simulink model "first"  (R2021a)
settings: Solver=FixedStepAuto  StartTime=0.0  StopTime=150  FixedStep=0.1  RelTol=1e-3
(part 1 of 2)
settings Model: Creator=templ  LastModifiedBy=templ
settings DataIOCC: ReturnWorkspaceOutputs=off

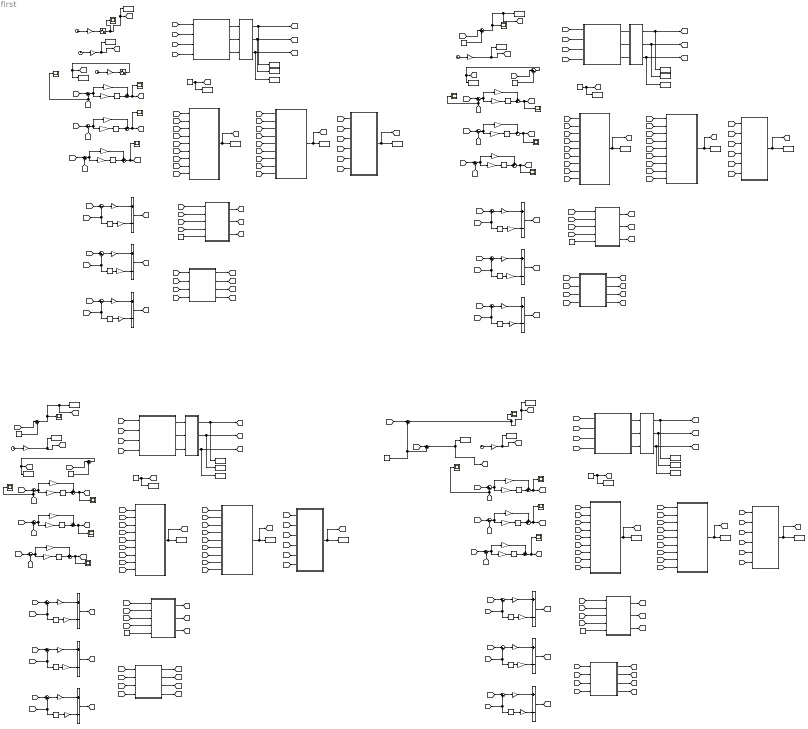
== system first ==
  note: Attitude
  note: Position
  note: Attitude
  note: Position
  note: Attitude
  note: Position
  note: Position
  note: Attitude
  Add{,1..11} (12 alike) : Sum  Inputs=+-
  Attitude Control Module : Subsystem
  Attitude Control Module1 : Subsystem
  Attitude Control Module2 : Subsystem
  Attitude Control Module3 : Subsystem
  Clock{,1..4,7} (6 alike) : Clock
  Constant{,1..4} (5 alike) : Constant  Value=5
  Derivative{,1..23} (24 alike) : Derivative
  Gain{,2,14,20,22,33,41,48} (8 alike) : Gain  Gain=0.03
  Gain{1,3,16,21,23,34,42,49} (8 alike) : Gain  Gain=0.8
  Gain{10,17,30,43} (4 alike) : Gain  Gain=0.25
  Gain{6,8,11,18,26,28,31,37,39,44,52,54} (12 alike) : Gain  Gain=0.5
  Gain{7,9,12..13,27,29,38,40,53,55} (10 alike) : Gain  Gain=0.2
  Gain{15,19,32,47} (4 alike) : Gain  Gain=0.1
  Gain{4,24,35,50} (4 alike) : Gain  Gain=0.05
  Gain{5,25,36,51} (4 alike) : Gain  Gain=0.32
  MATLAB Function : MATLAB Function  TreatAsAtomicUnit=on
  MATLAB Function1 : MATLAB Function  TreatAsAtomicUnit=on
  MATLAB Function2 : MATLAB Function  TreatAsAtomicUnit=on
  MATLAB Function3 : MATLAB Function  TreatAsAtomicUnit=on
  MATLAB Function4 : MATLAB Function  TreatAsAtomicUnit=on
  MATLAB Function5 : MATLAB Function  TreatAsAtomicUnit=on
  MATLAB Function6 : MATLAB Function  TreatAsAtomicUnit=on
  MATLAB Function7 : MATLAB Function  TreatAsAtomicUnit=on
  Position : MATLAB Function  TreatAsAtomicUnit=on
  Position1 : MATLAB Function  TreatAsAtomicUnit=on
  Position2 : MATLAB Function  TreatAsAtomicUnit=on
  Position3 : MATLAB Function  TreatAsAtomicUnit=on
  Scope{,1..19} (20 alike) : Scope
  Sine Wave : Sin  TimeSource=Use external signal  Amplitude=2  SampleTime=0
  Sine Wave Function1 : Sin  TimeSource=Use external signal  Amplitude=2  Phase=pi/2  SampleTime=0
  Subsystem : Subsystem
  Subsystem1 : Subsystem
  Subsystem2 : Subsystem
  Subsystem3 : Subsystem
  Subsystem4 : Subsystem
  Subsystem5 : Subsystem
  Subsystem6 : Subsystem
  Subsystem7 : Subsystem
  Sum{,2,4,6..9,11,13,15..19,21,23,25..27,30..31,33,35,37..39,41} (27 alike) : Sum  Inputs=|+-
  Sum{1,3,5,10,12,14,20,22,24,32,34,36} (12 alike) : Sum  Inputs=++|
  Sum28 : Sum  Inputs=|++
  Sum29 : Sum  Inputs=|++
  Sum40 : Sum  Inputs=|++
  To Workspace : ToWorkspace  VariableName=phi  SampleTime=-1
  To Workspace1 : ToWorkspace  VariableName=theta  SampleTime=-1
  To Workspace10 : ToWorkspace  VariableName=psaid  SampleTime=-1
  To Workspace11 : ToWorkspace  VariableName=theta1  SampleTime=-1
  To Workspace12 : ToWorkspace  VariableName=psaid1  SampleTime=-1
  To Workspace13 : ToWorkspace  VariableName=psai1  SampleTime=-1
  To Workspace14 : ToWorkspace  VariableName=x1  SampleTime=-1
  To Workspace15 : ToWorkspace  VariableName=y1  SampleTime=-1
  To Workspace16 : ToWorkspace  VariableName=z1  SampleTime=-1
  To Workspace17 : ToWorkspace  VariableName=xd1  SampleTime=-1
  To Workspace18 : ToWorkspace  VariableName=yd1  SampleTime=-1
  To Workspace19 : ToWorkspace  VariableName=zd1  SampleTime=-1
  To Workspace2 : ToWorkspace  VariableName=psai  SampleTime=-1
  To Workspace20 : ToWorkspace  VariableName=theta2  SampleTime=-1
  To Workspace21 : ToWorkspace  VariableName=psaid2  SampleTime=-1
  To Workspace22 : ToWorkspace  VariableName=psai2  SampleTime=-1
  To Workspace23 : ToWorkspace  VariableName=x2  SampleTime=-1
  To Workspace24 : ToWorkspace  VariableName=y2  SampleTime=-1
  To Workspace25 : ToWorkspace  VariableName=z2  SampleTime=-1
  To Workspace26 : ToWorkspace  VariableName=xd2  SampleTime=-1
  To Workspace27 : ToWorkspace  VariableName=yd2  SampleTime=-1
  To Workspace28 : ToWorkspace  VariableName=zd2  SampleTime=-1
  To Workspace29 : ToWorkspace  VariableName=phi2  SampleTime=-1
  To Workspace3 : ToWorkspace  VariableName=x  SampleTime=-1
  To Workspace30 : ToWorkspace  VariableName=phi3  SampleTime=-1
  To Workspace31 : ToWorkspace  VariableName=theta3  SampleTime=-1
  To Workspace32 : ToWorkspace  VariableName=psaid3  SampleTime=-1
  To Workspace33 : ToWorkspace  VariableName=psai3  SampleTime=-1
  To Workspace34 : ToWorkspace  VariableName=x3  SampleTime=-1
  To Workspace35 : ToWorkspace  VariableName=y3  SampleTime=-1
  To Workspace36 : ToWorkspace  VariableName=z3  SampleTime=-1
  To Workspace37 : ToWorkspace  VariableName=xd3  SampleTime=-1
  To Workspace38 : ToWorkspace  VariableName=yd3  SampleTime=-1
  To Workspace39 : ToWorkspace  VariableName=zd3  SampleTime=-1
  To Workspace4 : ToWorkspace  VariableName=y  SampleTime=-1
  To Workspace5 : ToWorkspace  VariableName=z  SampleTime=-1
  To Workspace6 : ToWorkspace  VariableName=xd  SampleTime=-1
  To Workspace7 : ToWorkspace  VariableName=yd  SampleTime=-1
  To Workspace8 : ToWorkspace  VariableName=zd  SampleTime=-1
  To Workspace9 : ToWorkspace  VariableName=phi1  SampleTime=-1
  m{,1..3} (4 alike) : Constant  Value=1.5
  psaid{1..4} (4 alike) : Constant  Value=0.2
  x : Subsystem
  x1 : Subsystem
  x2 : Subsystem
  x3 : Subsystem
  wires:
  Gain12/1 -> Sine Wave/1
  Sine Wave/1 -> Scope2/1, To Workspace6/1, [xd]
  Clock/1 -> Gain12/1
  Clock3/1 -> Gain15/1
  Gain15/1 -> [zd], To Workspace8/1
  Gain13/1 -> Sine Wave Function1/1
  Clock1/1 -> Gain13/1
  Sine Wave Function1/1 -> To Workspace7/1, [yd]
  Gain/1 -> Sum1/1
  Gain1/1 -> Derivative/1
  [x] -> Scope8/1, Sum/2
  Sum1/1 -> Scope/1, [Ux]
  Derivative/1 -> Sum1/2
  Sum/1 -> Gain1/1, Gain/1
  [xd] -> Sum/1
  Sum2/1 -> Gain3/1, Gain2/1
  Gain3/1 -> Derivative1/1
  Gain2/1 -> Sum3/1
  [y] -> Sum2/2
  Derivative1/1 -> Sum3/2
  [yd] -> Sum2/1
  [z] -> Sum4/2
  Sum4/1 -> Gain5/1, Gain4/1
  Gain4/1 -> Sum5/1
  [zd] -> Sum4/1
  Derivative2/1 -> Sum5/2
  Gain5/1 -> Derivative2/1
  [w2] -> Attitude Control Module/2(w2)
  [w1] -> Attitude Control Module/4(w1)
  [w3] -> Attitude Control Module/3(w3)
  MATLAB Function1/1(phi) -> To Workspace/1, [phi]
  MATLAB Function1/2(theta) -> To Workspace1/1, [theta]
  MATLAB Function1/3(psai) -> To Workspace2/1, [psai]
  Attitude Control Module/3(psai) -> MATLAB Function1/3(u3)
  Attitude Control Module/2(theta) -> MATLAB Function1/2(u2)
  Attitude Control Module/1(phi) -> MATLAB Function1/1(u1)
  [w4] -> Attitude Control Module/1(w4)
  [w4] -> Subsystem1/3(In3)
  [phi] -> Subsystem1/1(In1)
  [w3] -> Subsystem1/5(In5)
  [psai] -> Subsystem/3(In3)
  [theta] -> Subsystem/2(In2)
  [psai] -> x/3(In3)
  [w2] -> x/7(In7)
  [w4] -> x/6(In6)
  [theta] -> Subsystem1/2(In2)
  [phi] -> x/4(In4)
  [psai] -> x/5(In5)
  [w3] -> x/8(In8)
  [phi] -> Subsystem/4(In4)
  [w1] -> Subsystem1/6(In6)
  [w1] -> x/9(In9)
  [w1] -> Subsystem/9(In9)
  [psai] -> Subsystem/5(In5)
  [theta] -> x/2(In2)
  [w2] -> Subsystem/7(In7)
  [w4] -> Subsystem/6(In6)
  Subsystem1/1(Out1) -> [z], To Workspace5/1
  [w2] -> Subsystem1/4(In4)
  Subsystem/1(Out1) -> [y], To Workspace4/1
  [w3] -> Subsystem/8(In8)
  [phi] -> Subsystem/1(In1)
  x/1(Out1) -> [x], To Workspace3/1
  [phi] -> x/1(In1)
  Position/2(phid) -> [phid]
  Position/1(U1) -> [U1]
  [Uy] -> Position/2(Uy)
  [Ux] -> Position/1(Ux)
  m/1 -> Position/5(m)
  [psaid] -> Position/4(psaid)
  Position/3(thetad) -> [thetad]
  [Uz] -> Position/3(Uz)
  Gain7/1 -> Add/2
  Derivative3/1 -> Gain7/1
  [phid] -> Sum6/1
  [phi] -> Derivative3/1, Sum6/2
  Add/1 -> [U2]
  Gain6/1 -> Add/1
  Sum6/1 -> Gain6/1
  [theta] -> Derivative4/1, Sum7/2
  [thetad] -> Sum7/1
  Gain8/1 -> Add1/1
  Gain9/1 -> Add1/2
  Sum7/1 -> Gain8/1
  Derivative4/1 -> Gain9/1
  Add1/1 -> [U3]
  Derivative5/1 -> Gain11/1
  [psaid] -> Sum8/1
  Sum8/1 -> Gain10/1
  Gain10/1 -> Add2/1
  [psai] -> Derivative5/1, Sum8/2
  Add2/1 -> [U4]
  Gain11/1 -> Add2/2
  MATLAB Function/2(w2) -> [w2]
  MATLAB Function/3(w3) -> [w3]
  MATLAB Function/4(w4) -> [w4]
  MATLAB Function/1(w1) -> [w1]
  [U1] -> MATLAB Function/1(U1)
  [U3] -> MATLAB Function/3(U3)
  [U2] -> MATLAB Function/2(U2)
  [U4] -> MATLAB Function/4(U4)
  psaid1/1 -> To Workspace10/1, [psaid]
  Add4/1 -> [U31]
  Derivative10/1 -> Gain29/1
  Gain29/1 -> Add4/2
  Sum16/1 -> Gain28/1
  [theta1] -> Derivative10/1, Sum16/2
  Gain18/1 -> Add5/2
  Add5/1 -> [U41]
  [psai1] -> Derivative11/1, Sum17/2
  Gain17/1 -> Add5/1
  Sum17/1 -> Gain17/1
  [psaid1] -> Sum17/1
  [w11] -> Subsystem3/6(In6)
  [w21] -> Subsystem3/4(In4)
  Subsystem3/1(Out1) -> [z1], To Workspace16/1
  Derivative11/1 -> Gain18/1
  [w41] -> Subsystem2/6(In6)
  [w21] -> Subsystem2/7(In7)
  [theta1] -> x1/2(In2)
  [psai1] -> Subsystem2/5(In5)
  [w11] -> Subsystem2/9(In9)
  [w11] -> x1/9(In9)
  [phid1] -> Sum15/1
  Derivative9/1 -> Gain27/1
  [phi1] -> Derivative9/1, Sum15/2
  Add3/1 -> [U21]
  [U41] -> MATLAB Function2/4(U4)
  MATLAB Function2/4(w4) -> [w41]
  Gain16/1 -> Derivative6/1
  Gain14/1 -> Sum10/1
  [x1] -> Scope9/1, Sum9/2
  [phi1] -> Subsystem2/4(In4)
  Gain28/1 -> Add4/1
  psaid2/1 -> To Workspace12/1, [psaid1]
  [U21] -> MATLAB Function2/2(U2)
  [U11] -> MATLAB Function2/1(U1)
  [w31] -> x1/8(In8)
  MATLAB Function2/1(w1) -> [w11]
  m1/1 -> Position1/5(m)
  [Uz1] -> Position1/3(Uz)
  Position1/3(thetad) -> [thetad1]
  [psaid1] -> Position1/4(psaid)
  [w41] -> Subsystem3/3(In3)
  [Ux1] -> Position1/1(Ux)
  [xd1] -> Sum9/1
  Sum9/1 -> Gain16/1, Gain14/1
  Derivative6/1 -> Sum10/2
  [w31] -> Attitude Control Module1/3(w3)
  [w11] -> Attitude Control Module1/4(w1)
  MATLAB Function3/3(psai) -> To Workspace13/1, [psai1]
  [w21] -> Attitude Control Module1/2(w2)
  Attitude Control Module1/2(theta) -> MATLAB Function3/2(u2)
  Attitude Control Module1/3(psai) -> MATLAB Function3/3(u3)
  [Uy1] -> Position1/2(Uy)
  Gain27/1 -> Add3/2
  Position1/2(phid) -> [phid1]
  x1/1(Out1) -> [x1], To Workspace14/1
  [phi1] -> Subsystem2/1(In1)
  Gain26/1 -> Add3/1
  [phi1] -> x1/1(In1)
  Derivative8/1 -> Sum14/2
  Subsystem2/1(Out1) -> [y1], To Workspace15/1
  [thetad1] -> Sum16/1
  [zd1] -> Sum13/1
  Gain24/1 -> Sum14/1
  Attitude Control Module1/1(phi) -> MATLAB Function3/1(u1)
  [theta1] -> Subsystem3/2(In2)
  [w41] -> x1/6(In6)
  [U31] -> MATLAB Function2/3(U3)
  [w21] -> x1/7(In7)
  [w41] -> Attitude Control Module1/1(w4)
  MATLAB Function2/3(w3) -> [w31]
  [psai1] -> x1/3(In3)
  [theta1] -> Subsystem2/2(In2)
  [psai1] -> Subsystem2/3(In3)
  [w31] -> Subsystem3/5(In5)
  Sum13/1 -> Gain25/1, Gain24/1
  [psai1] -> x1/5(In5)
  MATLAB Function3/1(phi) -> To Workspace9/1, [phi1]
  [y1] -> Sum11/2
  Gain19/1 -> [zd1], To Workspace19/1
  [phi1] -> Subsystem3/1(In1)
  [w31] -> Subsystem2/8(In8)
  MATLAB Function3/2(theta) -> To Workspace11/1, [theta1]
  [yd1] -> Sum11/1
  Derivative7/1 -> Sum12/2
  Sum11/1 -> Gain23/1, Gain22/1
  [z1] -> Sum13/2
  Gain25/1 -> Derivative8/1
  MATLAB Function2/2(w2) -> [w21]
  [phi1] -> x1/4(In4)
  Gain23/1 -> Derivative7/1
  Position1/1(U1) -> [U11]
  Sum15/1 -> Gain26/1
  Gain22/1 -> Sum12/1
  [xd] -> Sum18/1
  Clock2/1 -> Gain19/1
  Sum3/1 -> Scope3/1, [Uy]
  Sum5/1 -> Scope4/1, [Uz]
  Sum10/1 -> Scope5/1, [Ux1]
  Sum12/1 -> Scope6/1, [Uy1]
  Sum14/1 -> Scope7/1, [Uz1]
  Constant/1 -> Sum18/2
  Sum18/1 -> Scope1/1, [xd1], To Workspace17/1
  Constant1/1 -> Sum19/2
  [yd] -> Sum19/1
  Sum19/1 -> To Workspace18/1, [yd1]
  [yd] -> Sum29/1
  Constant2/1 -> Sum28/2
  Clock4/1 -> Gain32/1
  [xd] -> Sum28/1
  Gain32/1 -> [zd2], To Workspace28/1
  Sum28/1 -> Scope10/1, [xd2], To Workspace26/1
  Sum29/1 -> To Workspace27/1, [yd2]
  [theta2] -> x2/2(In2)
  [w42] -> Subsystem4/6(In6)
  [w22] -> Subsystem5/4(In4)
  Add8/1 -> [U42]
  [psaid2] -> Sum27/1
  Derivative13/1 -> Gain31/1
  [w32] -> x2/8(In8)
  Sum23/1 -> Gain36/1, Gain35/1
  [yd2] -> Sum21/1
  MATLAB Function5/1(phi) -> To Workspace29/1, [phi2]
  [psai2] -> x2/5(In5)
  [phi2] -> x2/1(In1)
  MATLAB Function5/3(psai) -> To Workspace22/1, [psai2]
  [phi2] -> Subsystem5/1(In1)
  [w32] -> Subsystem5/5(In5)
  m2/1 -> Position2/5(m)
  Gain30/1 -> Add8/1
  Add6/1 -> [U22]
  [psai2] -> Subsystem4/3(In3)
  [theta2] -> Derivative12/1, Sum26/2
  [psai2] -> Subsystem4/5(In5)
  [psai2] -> x2/3(In3)
  MATLAB Function4/1(w1) -> [w12]
  [theta2] -> Subsystem4/2(In2)
  Sum24/1 -> Scope13/1, [Uz2]
  [w12] -> Subsystem5/6(In6)
  x2/1(Out1) -> [x2], To Workspace23/1
  [U32] -> MATLAB Function4/3(U3)
  Sum26/1 -> Gain39/1
  Gain38/1 -> Add6/2
  [thetad2] -> Sum26/1
  Sum20/1 -> Scope11/1, [Ux2]
  [psaid2] -> Position2/4(psaid)
  [zd2] -> Sum23/1
  [x2] -> Scope14/1, Sum30/2
  [theta2] -> Subsystem5/2(In2)
  Constant3/1 -> Sum29/2
  Attitude Control Module2/1(phi) -> MATLAB Function5/1(u1)
  [w12] -> Subsystem4/9(In9)
  Subsystem4/1(Out1) -> [y2], To Workspace24/1
  Attitude Control Module2/2(theta) -> MATLAB Function5/2(u2)
  Position2/3(thetad) -> [thetad2]
  [Ux2] -> Position2/1(Ux)
  Gain39/1 -> Add7/1
  Derivative17/1 -> Gain38/1
  Derivative12/1 -> Gain40/1
  [w12] -> Attitude Control Module2/4(w1)
  Position2/2(phid) -> [phid2]
  [xd2] -> Sum30/1
  [phid2] -> Sum25/1
  Attitude Control Module2/3(psai) -> MATLAB Function5/3(u3)
  MATLAB Function4/4(w4) -> [w42]
  [Uz2] -> Position2/3(Uz)
  [U12] -> MATLAB Function4/1(U1)
  [U22] -> MATLAB Function4/2(U2)
  psaid3/1 -> To Workspace21/1, [psaid2]
  Gain31/1 -> Add8/2
  [phi2] -> Derivative17/1, Sum25/2
  Subsystem5/1(Out1) -> [z2], To Workspace25/1
  Gain40/1 -> Add7/2
  [w12] -> x2/9(In9)
  Sum25/1 -> Gain37/1
  [phi2] -> Subsystem4/4(In4)
  Derivative14/1 -> Sum20/2
  Derivative16/1 -> Sum24/2
  [w42] -> x2/6(In6)
  MATLAB Function5/2(theta) -> To Workspace20/1, [theta2]
  [phi2] -> x2/4(In4)
  MATLAB Function4/2(w2) -> [w22]
  Derivative15/1 -> Sum22/2
  [w32] -> Attitude Control Module2/3(w3)
  Gain35/1 -> Sum24/1
  Add7/1 -> [U32]
  Sum30/1 -> Gain21/1, Gain20/1
  [w22] -> Subsystem4/7(In7)
  [y2] -> Sum21/2
  Gain37/1 -> Add6/1
  Sum21/1 -> Gain34/1, Gain33/1
  [w32] -> Subsystem4/8(In8)
  [w42] -> Subsystem5/3(In3)
  Gain36/1 -> Derivative16/1
  [phi2] -> Subsystem4/1(In1)
  [U42] -> MATLAB Function4/4(U4)
  [z2] -> Sum23/2
  [w22] -> Attitude Control Module2/2(w2)
  [w42] -> Attitude Control Module2/1(w4)
  Position2/1(U1) -> [U12]
  [psai2] -> Derivative13/1, Sum27/2
  Sum22/1 -> Scope12/1, [Uy2]
  Gain34/1 -> Derivative15/1
  [Uy2] -> Position2/2(Uy)
  [w22] -> x2/7(In7)
  Gain33/1 -> Sum22/1
  Sum27/1 -> Gain30/1
  MATLAB Function4/3(w3) -> [w32]
  Gain21/1 -> Derivative14/1
  Gain20/1 -> Sum20/1
  [psaid3] -> Sum39/1
  Sum35/1 -> Gain51/1, Gain50/1
  [x3] -> Scope19/1, Sum31/2
  Gain41/1 -> Sum32/1
  MATLAB Function7/2(theta) -> To Workspace31/1, [theta3]
  [theta3] -> Subsystem6/2(In2)
  Gain53/1 -> Add9/2
  Sum32/1 -> Scope15/1, [Ux3]
  [phi3] -> x3/1(In1)
  [psaid3] -> Position3/4(psaid)
  Clock7/1 -> Gain47/1
  MATLAB Function6/1(w1) -> [w13]
  [Uz3] -> Position3/3(Uz)
  Sum31/1 -> Gain42/1, Gain41/1
  Position3/3(thetad) -> [thetad3]
  [w33] -> Subsystem7/5(In5)
  m3/1 -> Position3/5(m)
  [w13] -> Subsystem6/9(In9)
  [Ux3] -> Position3/1(Ux)
  [w23] -> Subsystem6/7(In7)
  [phi3] -> x3/4(In4)
  [w23] -> Subsystem7/4(In4)
  [phi3] -> Subsystem6/4(In4)
  [psai3] -> x3/5(In5)
  [phid3] -> Sum37/1
  [psai3] -> Subsystem6/5(In5)
  [w43] -> Attitude Control Module3/1(w4)
  [w33] -> Attitude Control Module3/3(w3)
  [psai3] -> x3/3(In3)
  Gain51/1 -> Derivative20/1
  [w43] -> Subsystem7/3(In3)
  [w23] -> Attitude Control Module3/2(w2)
  MATLAB Function7/3(psai) -> To Workspace33/1, [psai3]
  Attitude Control Module3/1(phi) -> MATLAB Function7/1(u1)
  Derivative20/1 -> Sum36/2
  [w43] -> x3/6(In6)
  Gain50/1 -> Sum36/1
  [psai3] -> Subsystem6/3(In3)
  [w23] -> x3/7(In7)
  Derivative18/1 -> Sum32/2
  [y3] -> Sum33/2
  Gain48/1 -> Sum34/1
  [xd3] -> Sum31/1
  [z3] -> Sum35/2
  [yd3] -> Sum33/1
  Sum37/1 -> Gain52/1
  Gain44/1 -> Add11/2
  [psai3] -> Derivative23/1, Sum39/2
  Gain43/1 -> Add11/1
  x3/1(Out1) -> [x3], To Workspace34/1
  Gain54/1 -> Add10/1
  Attitude Control Module3/2(theta) -> MATLAB Function7/2(u2)
  [theta3] -> Derivative22/1, Sum38/2
  MATLAB Function7/1(phi) -> To Workspace30/1, [phi3]
  Add9/1 -> [U23]
  [w33] -> Subsystem6/8(In8)
  Gain52/1 -> Add9/1
  [phi3] -> Derivative21/1, Sum37/2
  Attitude Control Module3/3(psai) -> MATLAB Function7/3(u3)
  [w13] -> x3/9(In9)
  [phi3] -> Subsystem6/1(In1)
  [U33] -> MATLAB Function6/3(U3)
  Add11/1 -> [U43]
  [w43] -> Subsystem6/6(In6)
  MATLAB Function6/2(w2) -> [w23]
  [U23] -> MATLAB Function6/2(U2)
  [w33] -> x3/8(In8)
  psaid4/1 -> To Workspace32/1, [psaid3]
  MATLAB Function6/4(w4) -> [w43]
  Sum33/1 -> Gain49/1, Gain48/1
  Derivative19/1 -> Sum34/2
  Gain49/1 -> Derivative19/1
  Derivative21/1 -> Gain53/1
  [theta3] -> Subsystem7/2(In2)
  Gain47/1 -> [zd3], To Workspace39/1
  Derivative22/1 -> Gain55/1
  Sum41/1 -> [yd3], To Workspace38/1
  [w13] -> Attitude Control Module3/4(w1)
  MATLAB Function6/3(w3) -> [w33]
  [Uy3] -> Position3/2(Uy)
  Subsystem6/1(Out1) -> [y3], To Workspace35/1
  Gain55/1 -> Add10/2
  Subsystem7/1(Out1) -> [z3], To Workspace36/1
  Position3/1(U1) -> [U13]
  [w13] -> Subsystem7/6(In6)
  [zd3] -> Sum35/1
  [phi3] -> Subsystem7/1(In1)
  [U13] -> MATLAB Function6/1(U1)
  Derivative23/1 -> Gain44/1
  Add10/1 -> [U33]
  Sum39/1 -> Gain43/1
  [theta3] -> x3/2(In2)
  [U43] -> MATLAB Function6/4(U4)
  Sum36/1 -> Scope18/1, [Uz3]
  Gain42/1 -> Derivative18/1
  [thetad3] -> Sum38/1
  Sum34/1 -> Scope17/1, [Uy3]
  Sum38/1 -> Gain54/1
  Sum40/1 -> To Workspace37/1, [xd3], Scope16/1
  Position3/2(phid) -> [phid3]
  Constant4/1 -> Sum41/2, Sum40/2
  [x] -> Sum40/1
  [y] -> Sum41/1

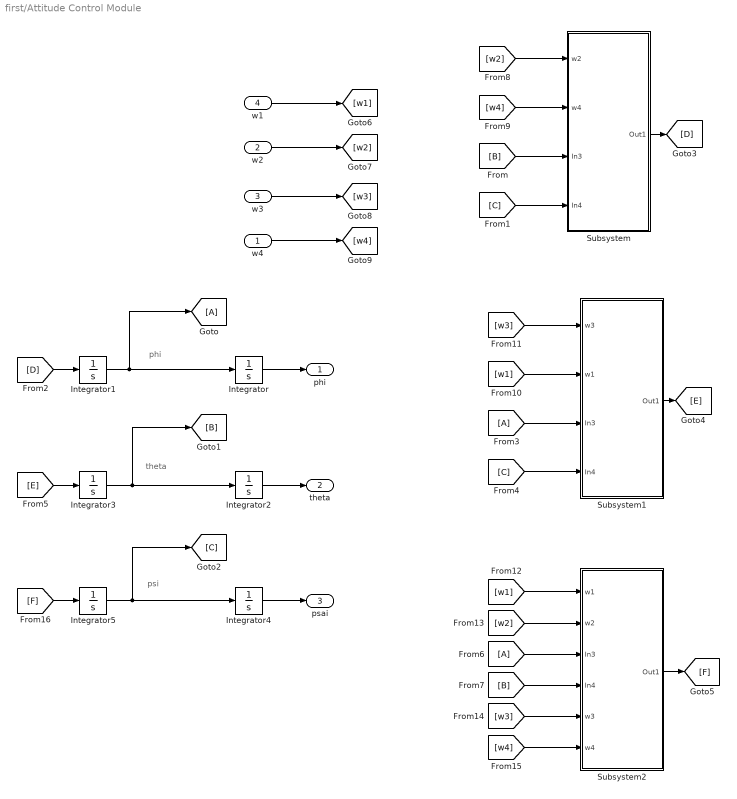
== system first/Attitude Control Module ==
  note: phi
  note: theta
  note: psi
  w4 : Inport
  w2 : Inport  Port=2
  w3 : Inport  Port=3
  w1 : Inport  Port=4
  Integrator{,1..5} (6 alike) : Integrator
  Subsystem : Subsystem
  Subsystem1 : Subsystem
  Subsystem2 : Subsystem
  phi : Outport  VectorParamsAs1DForOutWhenUnconnected=off
  theta : Outport  Port=2  VectorParamsAs1DForOutWhenUnconnected=off
  psai : Outport  Port=3  VectorParamsAs1DForOutWhenUnconnected=off
  wires:
  [w2] -> Subsystem2/2(w2)
  [D] -> Integrator1/1
  [w1] -> Subsystem2/1(w1)
  Integrator1/1 -> [A], Integrator/1
  Subsystem2/1(Out1) -> [F]
  [C] -> Subsystem1/4(In4)
  [B] -> Subsystem2/4(In4)
  [A] -> Subsystem2/3(In3)
  Integrator3/1 -> [B], Integrator2/1
  [A] -> Subsystem1/3(In3)
  [C] -> Subsystem/4(In4)
  Subsystem1/1(Out1) -> [E]
  [w4] -> Subsystem2/6(w4)
  [F] -> Integrator5/1
  [w2] -> Subsystem/1(w2)
  [w4] -> Subsystem/2(w4)
  [w3] -> Subsystem2/5(w3)
  Integrator2/1 -> theta/1
  Subsystem/1(Out1) -> [D]
  Integrator5/1 -> [C], Integrator4/1
  Integrator/1 -> phi/1
  Integrator4/1 -> psai/1
  w4/1 -> [w4]
  w2/1 -> [w2]
  [B] -> Subsystem/3(In3)
  [E] -> Integrator3/1
  w1/1 -> [w1]
  w3/1 -> [w3]
  [w3] -> Subsystem1/1(w3)
  [w1] -> Subsystem1/2(w1)

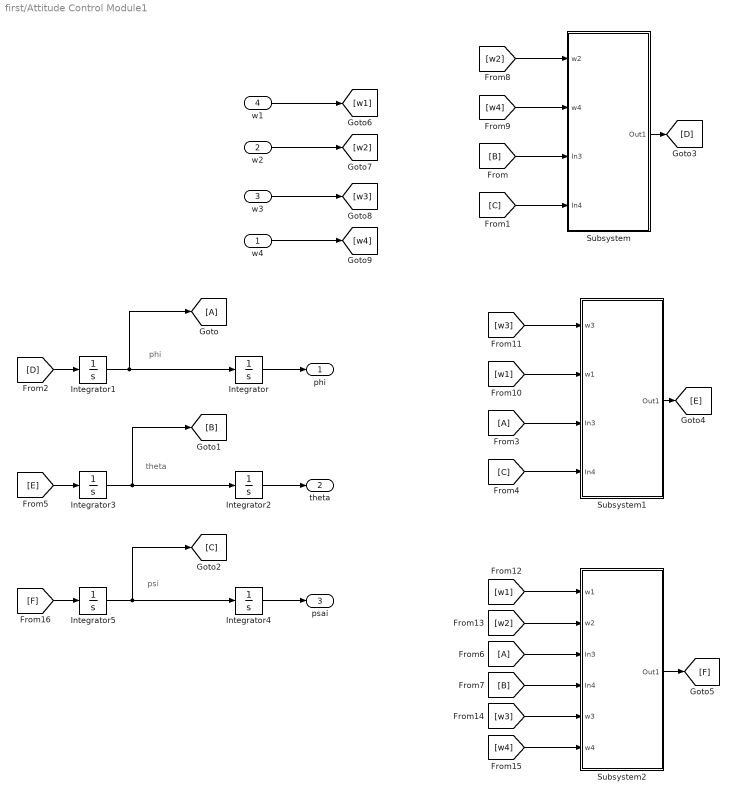
== system first/Attitude Control Module1 ==
  note: phi
  note: theta
  note: psi
  w4 : Inport
  w2 : Inport  Port=2
  w3 : Inport  Port=3
  w1 : Inport  Port=4
  Integrator{,1..5} (6 alike) : Integrator
  Subsystem : Subsystem
  Subsystem1 : Subsystem
  Subsystem2 : Subsystem
  phi : Outport  VectorParamsAs1DForOutWhenUnconnected=off
  theta : Outport  Port=2  VectorParamsAs1DForOutWhenUnconnected=off
  psai : Outport  Port=3  VectorParamsAs1DForOutWhenUnconnected=off
  wires:
  [w2] -> Subsystem2/2(w2)
  [D] -> Integrator1/1
  [w1] -> Subsystem2/1(w1)
  Integrator1/1 -> [A], Integrator/1
  Subsystem2/1(Out1) -> [F]
  [C] -> Subsystem1/4(In4)
  [B] -> Subsystem2/4(In4)
  [A] -> Subsystem2/3(In3)
  Integrator3/1 -> [B], Integrator2/1
  [A] -> Subsystem1/3(In3)
  [C] -> Subsystem/4(In4)
  Subsystem1/1(Out1) -> [E]
  [w4] -> Subsystem2/6(w4)
  [F] -> Integrator5/1
  [w2] -> Subsystem/1(w2)
  [w4] -> Subsystem/2(w4)
  [w3] -> Subsystem2/5(w3)
  Integrator2/1 -> theta/1
  Subsystem/1(Out1) -> [D]
  Integrator5/1 -> [C], Integrator4/1
  Integrator/1 -> phi/1
  Integrator4/1 -> psai/1
  w4/1 -> [w4]
  w2/1 -> [w2]
  [B] -> Subsystem/3(In3)
  [E] -> Integrator3/1
  w1/1 -> [w1]
  w3/1 -> [w3]
  [w3] -> Subsystem1/1(w3)
  [w1] -> Subsystem1/2(w1)

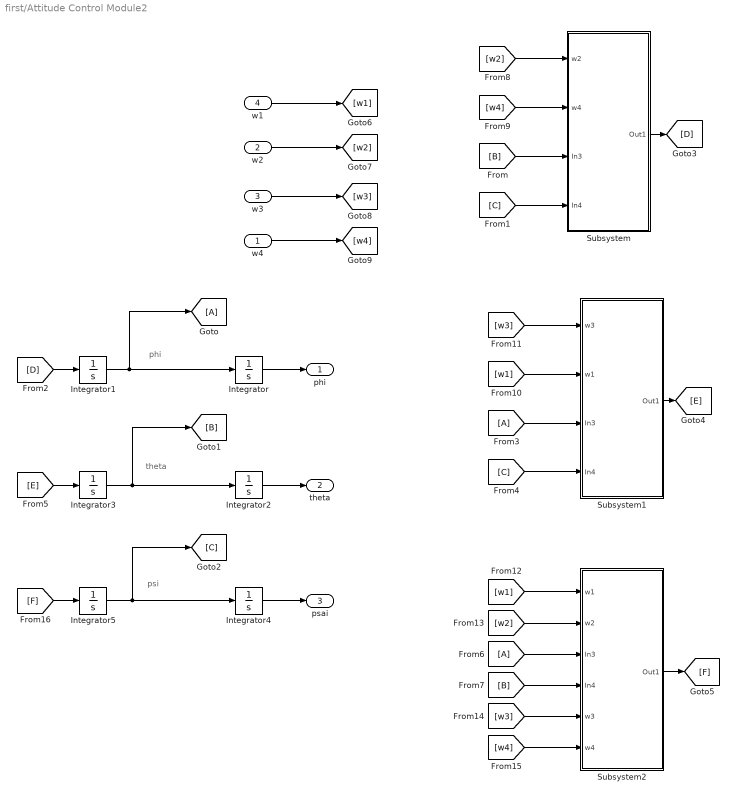
== system first/Attitude Control Module2 ==
  note: phi
  note: theta
  note: psi
  w4 : Inport
  w2 : Inport  Port=2
  w3 : Inport  Port=3
  w1 : Inport  Port=4
  Integrator{,1..5} (6 alike) : Integrator
  Subsystem : Subsystem
  Subsystem1 : Subsystem
  Subsystem2 : Subsystem
  phi : Outport  VectorParamsAs1DForOutWhenUnconnected=off
  theta : Outport  Port=2  VectorParamsAs1DForOutWhenUnconnected=off
  psai : Outport  Port=3  VectorParamsAs1DForOutWhenUnconnected=off
  wires:
  [w2] -> Subsystem2/2(w2)
  [D] -> Integrator1/1
  [w1] -> Subsystem2/1(w1)
  Integrator1/1 -> [A], Integrator/1
  Subsystem2/1(Out1) -> [F]
  [C] -> Subsystem1/4(In4)
  [B] -> Subsystem2/4(In4)
  [A] -> Subsystem2/3(In3)
  Integrator3/1 -> [B], Integrator2/1
  [A] -> Subsystem1/3(In3)
  [C] -> Subsystem/4(In4)
  Subsystem1/1(Out1) -> [E]
  [w4] -> Subsystem2/6(w4)
  [F] -> Integrator5/1
  [w2] -> Subsystem/1(w2)
  [w4] -> Subsystem/2(w4)
  [w3] -> Subsystem2/5(w3)
  Integrator2/1 -> theta/1
  Subsystem/1(Out1) -> [D]
  Integrator5/1 -> [C], Integrator4/1
  Integrator/1 -> phi/1
  Integrator4/1 -> psai/1
  w4/1 -> [w4]
  w2/1 -> [w2]
  [B] -> Subsystem/3(In3)
  [E] -> Integrator3/1
  w1/1 -> [w1]
  w3/1 -> [w3]
  [w3] -> Subsystem1/1(w3)
  [w1] -> Subsystem1/2(w1)

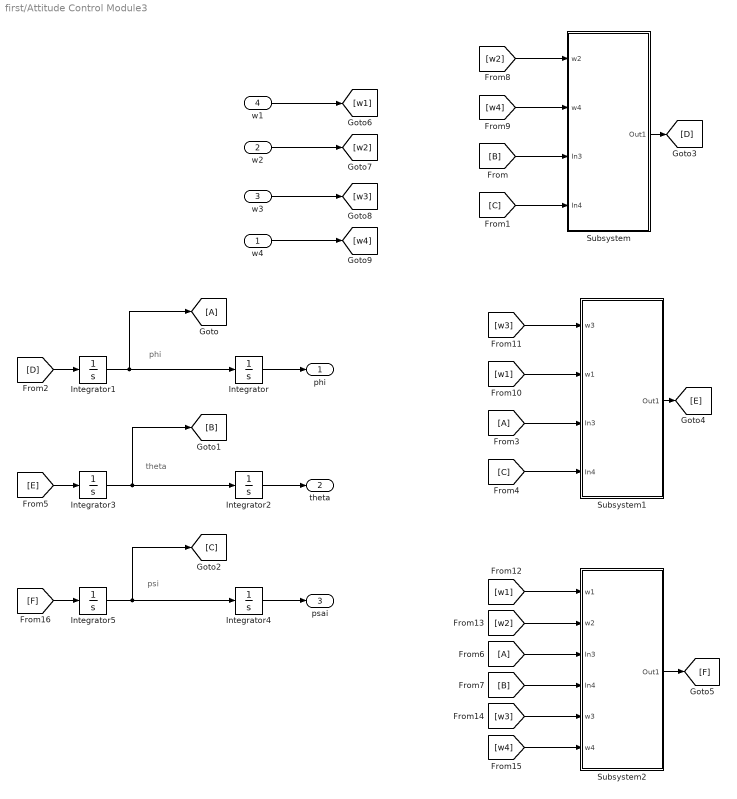
== system first/Attitude Control Module3 ==
  note: phi
  note: theta
  note: psi
  w4 : Inport
  w2 : Inport  Port=2
  w3 : Inport  Port=3
  w1 : Inport  Port=4
  Integrator{,1..5} (6 alike) : Integrator
  Subsystem : Subsystem
  Subsystem1 : Subsystem
  Subsystem2 : Subsystem
  phi : Outport  VectorParamsAs1DForOutWhenUnconnected=off
  theta : Outport  Port=2  VectorParamsAs1DForOutWhenUnconnected=off
  psai : Outport  Port=3  VectorParamsAs1DForOutWhenUnconnected=off
  wires:
  [w2] -> Subsystem2/2(w2)
  [D] -> Integrator1/1
  [w1] -> Subsystem2/1(w1)
  Integrator1/1 -> [A], Integrator/1
  Subsystem2/1(Out1) -> [F]
  [C] -> Subsystem1/4(In4)
  [B] -> Subsystem2/4(In4)
  [A] -> Subsystem2/3(In3)
  Integrator3/1 -> [B], Integrator2/1
  [A] -> Subsystem1/3(In3)
  [C] -> Subsystem/4(In4)
  Subsystem1/1(Out1) -> [E]
  [w4] -> Subsystem2/6(w4)
  [F] -> Integrator5/1
  [w2] -> Subsystem/1(w2)
  [w4] -> Subsystem/2(w4)
  [w3] -> Subsystem2/5(w3)
  Integrator2/1 -> theta/1
  Subsystem/1(Out1) -> [D]
  Integrator5/1 -> [C], Integrator4/1
  Integrator/1 -> phi/1
  Integrator4/1 -> psai/1
  w4/1 -> [w4]
  w2/1 -> [w2]
  [B] -> Subsystem/3(In3)
  [E] -> Integrator3/1
  w1/1 -> [w1]
  w3/1 -> [w3]
  [w3] -> Subsystem1/1(w3)
  [w1] -> Subsystem1/2(w1)

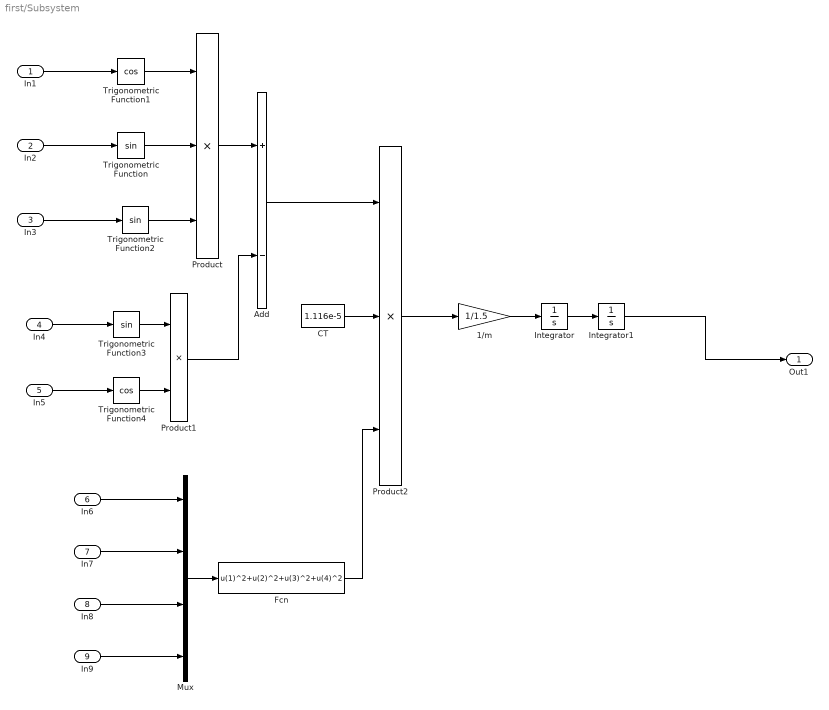
== system first/Subsystem ==
  In1 : Inport
  In2 : Inport  Port=2
  In3 : Inport  Port=3
  In4 : Inport  Port=4
  In5 : Inport  Port=5
  In6 : Inport  Port=6
  In7 : Inport  Port=7
  In8 : Inport  Port=8
  In9 : Inport  Port=9
  1/m : Gain  Gain=1/1.5
  Add : Sum  Inputs=+-
  CT : Constant  Value=1.116e-5
  Fcn : Fcn  Expr=u(1)^2+u(2)^2+u(3)^2+u(4)^2
  Integrator : Integrator
  Integrator1 : Integrator
  Mux : Mux
  Product : Product  Inputs=3
  Product1 : Product
  Product2 : Product  Inputs=3
  Trigonometric Function : Trigonometry
  Trigonometric Function1 : Trigonometry  Operator=cos
  Trigonometric Function2 : Trigonometry
  Trigonometric Function3 : Trigonometry
  Trigonometric Function4 : Trigonometry  Operator=cos
  Out1 : Outport  VectorParamsAs1DForOutWhenUnconnected=off
  wires:
  Mux/1 -> Fcn/1
  Product2/1 -> 1/m/1
  Fcn/1 -> Product2/3
  CT/1 -> Product2/2
  Trigonometric Function2/1 -> Product/3
  Trigonometric Function/1 -> Product/2
  Trigonometric Function3/1 -> Product1/1
  Product1/1 -> Add/2
  Product/1 -> Add/1
  Add/1 -> Product2/1
  In4/1 -> Trigonometric Function3/1
  Trigonometric Function1/1 -> Product/1
  Integrator/1 -> Integrator1/1
  In8/1 -> Mux/3
  Trigonometric Function4/1 -> Product1/2
  1/m/1 -> Integrator/1
  Integrator1/1 -> Out1/1
  In9/1 -> Mux/4
  In1/1 -> Trigonometric Function1/1
  In6/1 -> Mux/1
  In5/1 -> Trigonometric Function4/1
  In7/1 -> Mux/2
  In3/1 -> Trigonometric Function2/1
  In2/1 -> Trigonometric Function/1

== system first/Subsystem1 ==
  In1 : Inport
  In2 : Inport  Port=2
  In3 : Inport  Port=3
  In4 : Inport  Port=4
  In5 : Inport  Port=5
  In6 : Inport  Port=6
  1/m : Gain  Gain=1/1.5
  Add : Sum  Inputs=+-
  CT : Constant  Value=1.116e-5
  Fcn : Fcn  Expr=u(1)^2+u(2)^2+u(3)^2+u(4)^2
  Integrator : Integrator
  Integrator1 : Integrator
  Mux : Mux
  Product1 : Product  Inputs=4
  Trigonometric Function : Trigonometry  Operator=cos
  Trigonometric Function1 : Trigonometry  Operator=cos
  mg : Constant  Value=1.5*9.81
  Out1 : Outport  VectorParamsAs1DForOutWhenUnconnected=off
  wires:
  Trigonometric Function1/1 -> Product1/1
  Integrator/1 -> Integrator1/1
  Fcn/1 -> Product1/4
  mg/1 -> Add/2
  CT/1 -> Product1/3
  Add/1 -> 1/m/1
  Mux/1 -> Fcn/1
  In2/1 -> Trigonometric Function/1
  1/m/1 -> Integrator/1
  Trigonometric Function/1 -> Product1/2
  Product1/1 -> Add/1
  In4/1 -> Mux/2
  Integrator1/1 -> Out1/1
  In5/1 -> Mux/3
  In3/1 -> Mux/1
  In6/1 -> Mux/4
  In1/1 -> Trigonometric Function1/1

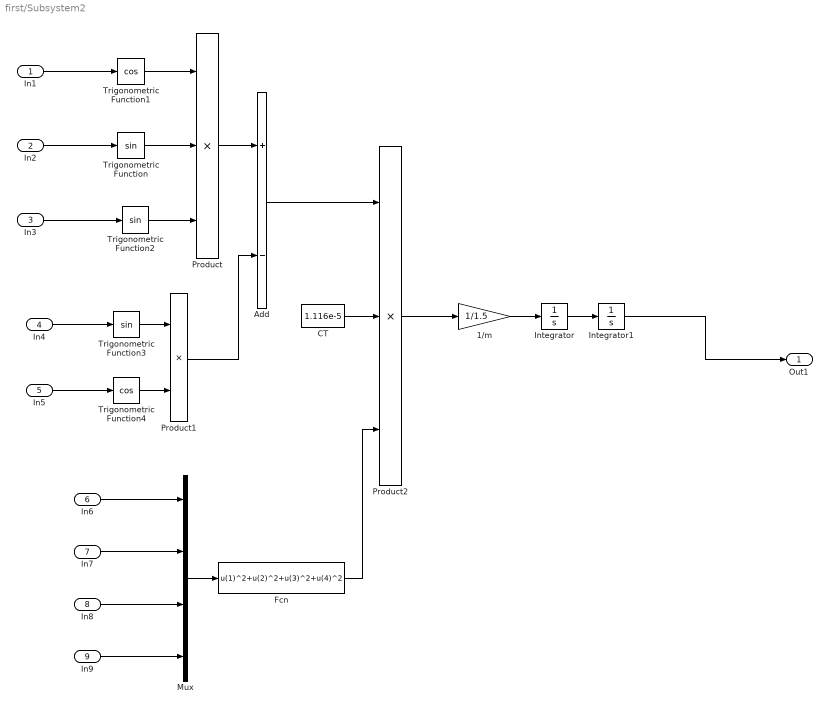
== system first/Subsystem2 ==
  In1 : Inport
  In2 : Inport  Port=2
  In3 : Inport  Port=3
  In4 : Inport  Port=4
  In5 : Inport  Port=5
  In6 : Inport  Port=6
  In7 : Inport  Port=7
  In8 : Inport  Port=8
  In9 : Inport  Port=9
  1/m : Gain  Gain=1/1.5
  Add : Sum  Inputs=+-
  CT : Constant  Value=1.116e-5
  Fcn : Fcn  Expr=u(1)^2+u(2)^2+u(3)^2+u(4)^2
  Integrator : Integrator
  Integrator1 : Integrator
  Mux : Mux
  Product : Product  Inputs=3
  Product1 : Product
  Product2 : Product  Inputs=3
  Trigonometric Function : Trigonometry
  Trigonometric Function1 : Trigonometry  Operator=cos
  Trigonometric Function2 : Trigonometry
  Trigonometric Function3 : Trigonometry
  Trigonometric Function4 : Trigonometry  Operator=cos
  Out1 : Outport  VectorParamsAs1DForOutWhenUnconnected=off
  wires:
  Mux/1 -> Fcn/1
  Product2/1 -> 1/m/1
  Fcn/1 -> Product2/3
  CT/1 -> Product2/2
  Trigonometric Function2/1 -> Product/3
  Trigonometric Function/1 -> Product/2
  Trigonometric Function3/1 -> Product1/1
  Product1/1 -> Add/2
  Product/1 -> Add/1
  Add/1 -> Product2/1
  In4/1 -> Trigonometric Function3/1
  Trigonometric Function1/1 -> Product/1
  Integrator/1 -> Integrator1/1
  In8/1 -> Mux/3
  Trigonometric Function4/1 -> Product1/2
  1/m/1 -> Integrator/1
  Integrator1/1 -> Out1/1
  In9/1 -> Mux/4
  In1/1 -> Trigonometric Function1/1
  In6/1 -> Mux/1
  In5/1 -> Trigonometric Function4/1
  In7/1 -> Mux/2
  In3/1 -> Trigonometric Function2/1
  In2/1 -> Trigonometric Function/1

== system first/Subsystem3 ==
  In1 : Inport
  In2 : Inport  Port=2
  In3 : Inport  Port=3
  In4 : Inport  Port=4
  In5 : Inport  Port=5
  In6 : Inport  Port=6
  1/m : Gain  Gain=1/1.5
  Add : Sum  Inputs=+-
  CT : Constant  Value=1.116e-5
  Fcn : Fcn  Expr=u(1)^2+u(2)^2+u(3)^2+u(4)^2
  Integrator : Integrator
  Integrator1 : Integrator
  Mux : Mux
  Product1 : Product  Inputs=4
  Trigonometric Function : Trigonometry  Operator=cos
  Trigonometric Function1 : Trigonometry  Operator=cos
  mg : Constant  Value=1.5*9.81
  Out1 : Outport  VectorParamsAs1DForOutWhenUnconnected=off
  wires:
  Trigonometric Function1/1 -> Product1/1
  Integrator/1 -> Integrator1/1
  Fcn/1 -> Product1/4
  mg/1 -> Add/2
  CT/1 -> Product1/3
  Add/1 -> 1/m/1
  Mux/1 -> Fcn/1
  In2/1 -> Trigonometric Function/1
  1/m/1 -> Integrator/1
  Trigonometric Function/1 -> Product1/2
  Product1/1 -> Add/1
  In4/1 -> Mux/2
  Integrator1/1 -> Out1/1
  In5/1 -> Mux/3
  In3/1 -> Mux/1
  In6/1 -> Mux/4
  In1/1 -> Trigonometric Function1/1

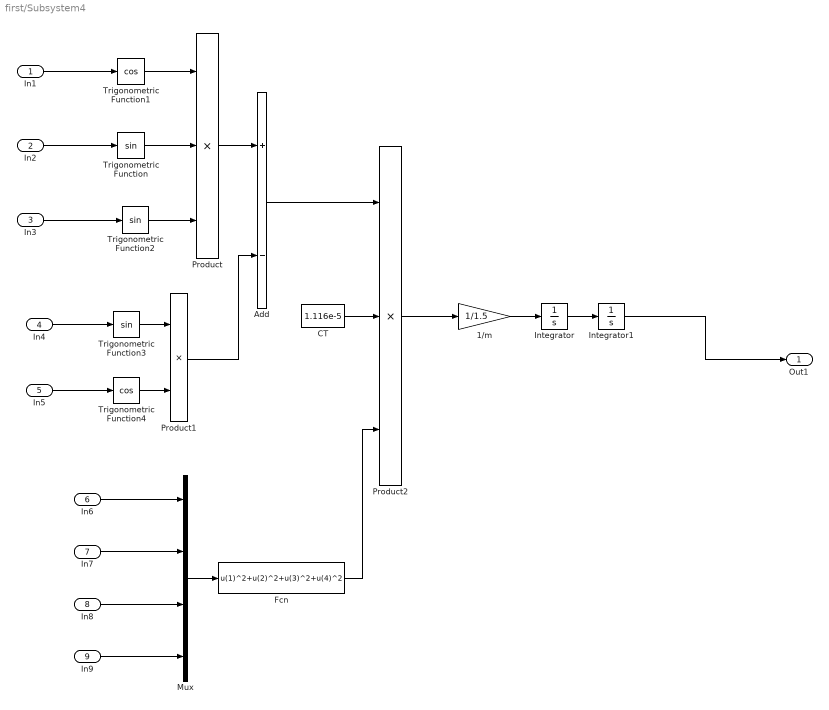
== system first/Subsystem4 ==
  In1 : Inport
  In2 : Inport  Port=2
  In3 : Inport  Port=3
  In4 : Inport  Port=4
  In5 : Inport  Port=5
  In6 : Inport  Port=6
  In7 : Inport  Port=7
  In8 : Inport  Port=8
  In9 : Inport  Port=9
  1/m : Gain  Gain=1/1.5
  Add : Sum  Inputs=+-
  CT : Constant  Value=1.116e-5
  Fcn : Fcn  Expr=u(1)^2+u(2)^2+u(3)^2+u(4)^2
  Integrator : Integrator
  Integrator1 : Integrator
  Mux : Mux
  Product : Product  Inputs=3
  Product1 : Product
  Product2 : Product  Inputs=3
  Trigonometric Function : Trigonometry
  Trigonometric Function1 : Trigonometry  Operator=cos
  Trigonometric Function2 : Trigonometry
  Trigonometric Function3 : Trigonometry
  Trigonometric Function4 : Trigonometry  Operator=cos
  Out1 : Outport  VectorParamsAs1DForOutWhenUnconnected=off
  wires:
  Mux/1 -> Fcn/1
  Product2/1 -> 1/m/1
  Fcn/1 -> Product2/3
  CT/1 -> Product2/2
  Trigonometric Function2/1 -> Product/3
  Trigonometric Function/1 -> Product/2
  Trigonometric Function3/1 -> Product1/1
  Product1/1 -> Add/2
  Product/1 -> Add/1
  Add/1 -> Product2/1
  In4/1 -> Trigonometric Function3/1
  Trigonometric Function1/1 -> Product/1
  Integrator/1 -> Integrator1/1
  In8/1 -> Mux/3
  Trigonometric Function4/1 -> Product1/2
  1/m/1 -> Integrator/1
  Integrator1/1 -> Out1/1
  In9/1 -> Mux/4
  In1/1 -> Trigonometric Function1/1
  In6/1 -> Mux/1
  In5/1 -> Trigonometric Function4/1
  In7/1 -> Mux/2
  In3/1 -> Trigonometric Function2/1
  In2/1 -> Trigonometric Function/1

== system first/Subsystem5 ==
  In1 : Inport
  In2 : Inport  Port=2
  In3 : Inport  Port=3
  In4 : Inport  Port=4
  In5 : Inport  Port=5
  In6 : Inport  Port=6
  1/m : Gain  Gain=1/1.5
  Add : Sum  Inputs=+-
  CT : Constant  Value=1.116e-5
  Fcn : Fcn  Expr=u(1)^2+u(2)^2+u(3)^2+u(4)^2
  Integrator : Integrator
  Integrator1 : Integrator
  Mux : Mux
  Product1 : Product  Inputs=4
  Trigonometric Function : Trigonometry  Operator=cos
  Trigonometric Function1 : Trigonometry  Operator=cos
  mg : Constant  Value=1.5*9.81
  Out1 : Outport  VectorParamsAs1DForOutWhenUnconnected=off
  wires:
  Trigonometric Function1/1 -> Product1/1
  Integrator/1 -> Integrator1/1
  Fcn/1 -> Product1/4
  mg/1 -> Add/2
  CT/1 -> Product1/3
  Add/1 -> 1/m/1
  Mux/1 -> Fcn/1
  In2/1 -> Trigonometric Function/1
  1/m/1 -> Integrator/1
  Trigonometric Function/1 -> Product1/2
  Product1/1 -> Add/1
  In4/1 -> Mux/2
  Integrator1/1 -> Out1/1
  In5/1 -> Mux/3
  In3/1 -> Mux/1
  In6/1 -> Mux/4
  In1/1 -> Trigonometric Function1/1

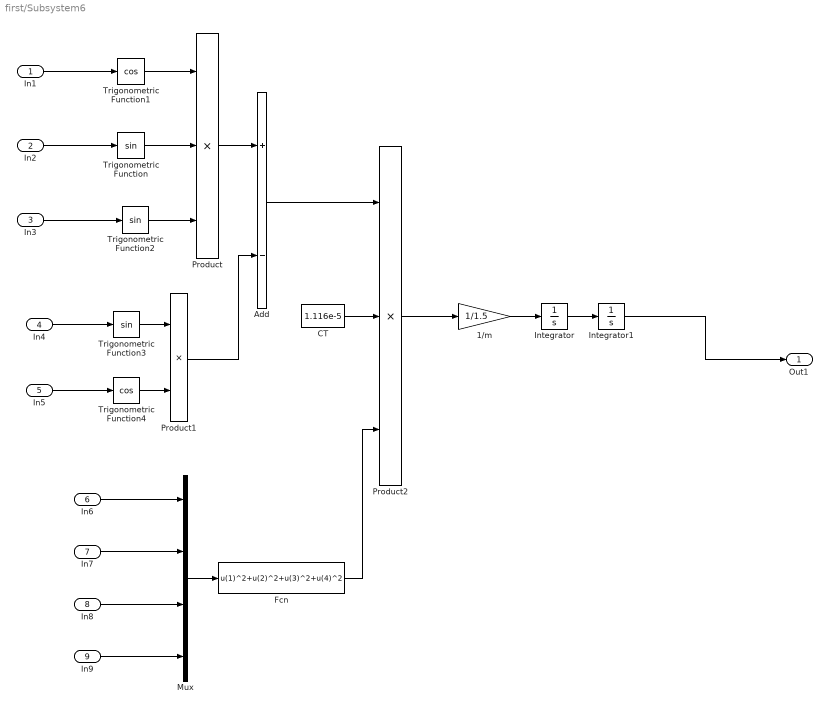
== system first/Subsystem6 ==
  In1 : Inport
  In2 : Inport  Port=2
  In3 : Inport  Port=3
  In4 : Inport  Port=4
  In5 : Inport  Port=5
  In6 : Inport  Port=6
  In7 : Inport  Port=7
  In8 : Inport  Port=8
  In9 : Inport  Port=9
  1/m : Gain  Gain=1/1.5
  Add : Sum  Inputs=+-
  CT : Constant  Value=1.116e-5
  Fcn : Fcn  Expr=u(1)^2+u(2)^2+u(3)^2+u(4)^2
  Integrator : Integrator
  Integrator1 : Integrator
  Mux : Mux
  Product : Product  Inputs=3
  Product1 : Product
  Product2 : Product  Inputs=3
  Trigonometric Function : Trigonometry
  Trigonometric Function1 : Trigonometry  Operator=cos
  Trigonometric Function2 : Trigonometry
  Trigonometric Function3 : Trigonometry
  Trigonometric Function4 : Trigonometry  Operator=cos
  Out1 : Outport  VectorParamsAs1DForOutWhenUnconnected=off
  wires:
  Mux/1 -> Fcn/1
  Product2/1 -> 1/m/1
  Fcn/1 -> Product2/3
  CT/1 -> Product2/2
  Trigonometric Function2/1 -> Product/3
  Trigonometric Function/1 -> Product/2
  Trigonometric Function3/1 -> Product1/1
  Product1/1 -> Add/2
  Product/1 -> Add/1
  Add/1 -> Product2/1
  In4/1 -> Trigonometric Function3/1
  Trigonometric Function1/1 -> Product/1
  Integrator/1 -> Integrator1/1
  In8/1 -> Mux/3
  Trigonometric Function4/1 -> Product1/2
  1/m/1 -> Integrator/1
  Integrator1/1 -> Out1/1
  In9/1 -> Mux/4
  In1/1 -> Trigonometric Function1/1
  In6/1 -> Mux/1
  In5/1 -> Trigonometric Function4/1
  In7/1 -> Mux/2
  In3/1 -> Trigonometric Function2/1
  In2/1 -> Trigonometric Function/1

== system first/Subsystem7 ==
  In1 : Inport
  In2 : Inport  Port=2
  In3 : Inport  Port=3
  In4 : Inport  Port=4
  In5 : Inport  Port=5
  In6 : Inport  Port=6
  1/m : Gain  Gain=1/1.5
  Add : Sum  Inputs=+-
  CT : Constant  Value=1.116e-5
  Fcn : Fcn  Expr=u(1)^2+u(2)^2+u(3)^2+u(4)^2
  Integrator : Integrator
  Integrator1 : Integrator
  Mux : Mux
  Product1 : Product  Inputs=4
  Trigonometric Function : Trigonometry  Operator=cos
  Trigonometric Function1 : Trigonometry  Operator=cos
  mg : Constant  Value=1.5*9.81
  Out1 : Outport  VectorParamsAs1DForOutWhenUnconnected=off
  wires:
  Trigonometric Function1/1 -> Product1/1
  Integrator/1 -> Integrator1/1
  Fcn/1 -> Product1/4
  mg/1 -> Add/2
  CT/1 -> Product1/3
  Add/1 -> 1/m/1
  Mux/1 -> Fcn/1
  In2/1 -> Trigonometric Function/1
  1/m/1 -> Integrator/1
  Trigonometric Function/1 -> Product1/2
  Product1/1 -> Add/1
  In4/1 -> Mux/2
  Integrator1/1 -> Out1/1
  In5/1 -> Mux/3
  In3/1 -> Mux/1
  In6/1 -> Mux/4
  In1/1 -> Trigonometric Function1/1

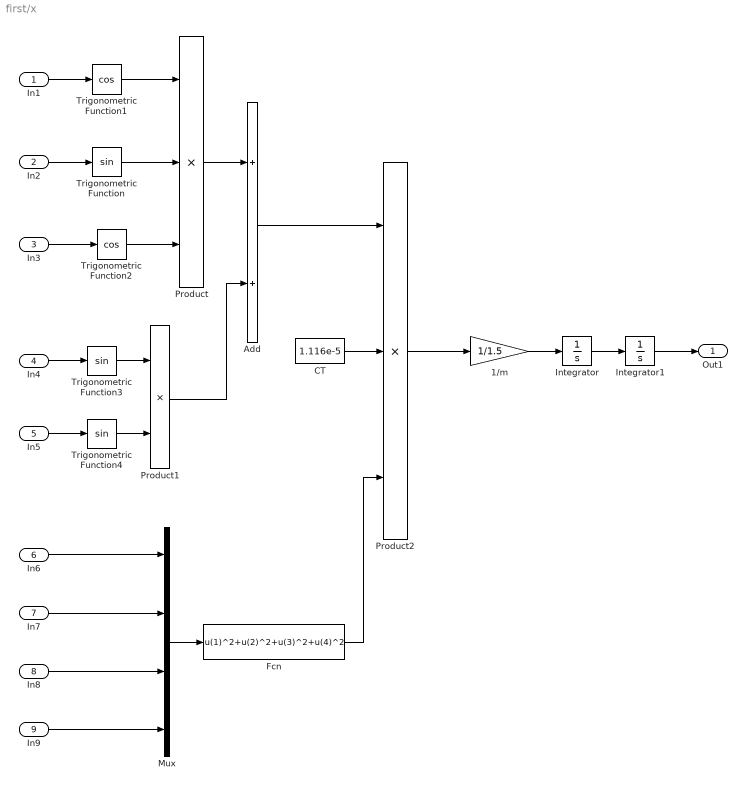
== system first/x ==
  In1 : Inport
  In2 : Inport  Port=2
  In3 : Inport  Port=3
  In4 : Inport  Port=4
  In5 : Inport  Port=5
  In6 : Inport  Port=6
  In7 : Inport  Port=7
  In8 : Inport  Port=8
  In9 : Inport  Port=9
  1/m : Gain  Gain=1/1.5
  Add : Sum
  CT : Constant  Value=1.116e-5
  Fcn : Fcn  Expr=u(1)^2+u(2)^2+u(3)^2+u(4)^2
  Integrator : Integrator
  Integrator1 : Integrator
  Mux : Mux
  Product : Product  Inputs=3
  Product1 : Product
  Product2 : Product  Inputs=3
  Trigonometric Function : Trigonometry
  Trigonometric Function1 : Trigonometry  Operator=cos
  Trigonometric Function2 : Trigonometry  Operator=cos
  Trigonometric Function3 : Trigonometry
  Trigonometric Function4 : Trigonometry
  Out1 : Outport  VectorParamsAs1DForOutWhenUnconnected=off
  wires:
  In8/1 -> Mux/3
  Integrator1/1 -> Out1/1
  1/m/1 -> Integrator/1
  Trigonometric Function4/1 -> Product1/2
  Integrator/1 -> Integrator1/1
  In7/1 -> Mux/2
  Add/1 -> Product2/1
  Product1/1 -> Add/2
  Product/1 -> Add/1
  In4/1 -> Trigonometric Function3/1
  Fcn/1 -> Product2/3
  Trigonometric Function1/1 -> Product/1
  In2/1 -> Trigonometric Function/1
  Trigonometric Function/1 -> Product/2
  Trigonometric Function2/1 -> Product/3
  Trigonometric Function3/1 -> Product1/1
  CT/1 -> Product2/2
  In1/1 -> Trigonometric Function1/1
  Product2/1 -> 1/m/1
  In3/1 -> Trigonometric Function2/1
  Mux/1 -> Fcn/1
  In6/1 -> Mux/1
  In5/1 -> Trigonometric Function4/1
  In9/1 -> Mux/4

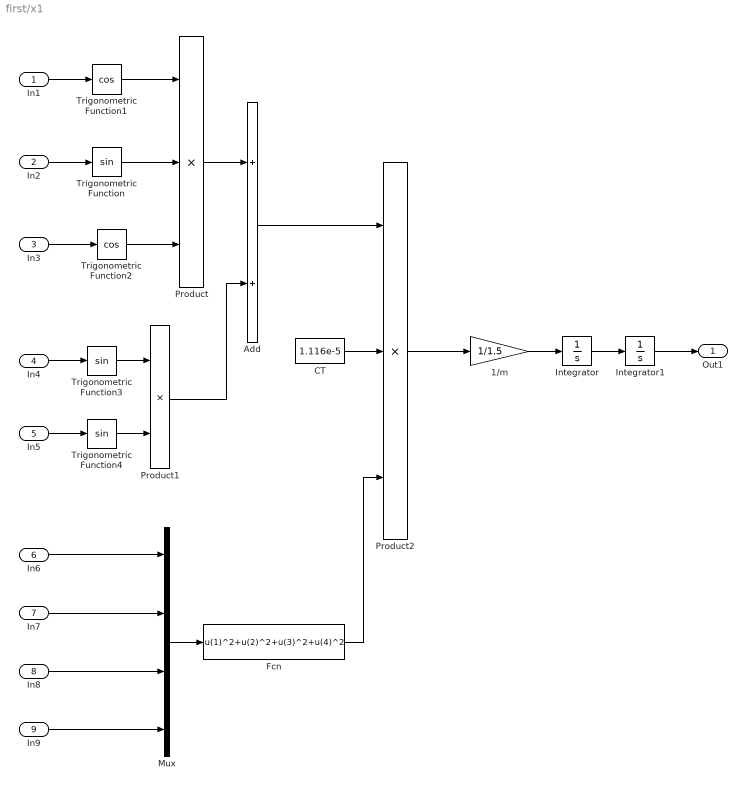
== system first/x1 ==
  In1 : Inport
  In2 : Inport  Port=2
  In3 : Inport  Port=3
  In4 : Inport  Port=4
  In5 : Inport  Port=5
  In6 : Inport  Port=6
  In7 : Inport  Port=7
  In8 : Inport  Port=8
  In9 : Inport  Port=9
  1/m : Gain  Gain=1/1.5
  Add : Sum
  CT : Constant  Value=1.116e-5
  Fcn : Fcn  Expr=u(1)^2+u(2)^2+u(3)^2+u(4)^2
  Integrator : Integrator
  Integrator1 : Integrator
  Mux : Mux
  Product : Product  Inputs=3
  Product1 : Product
  Product2 : Product  Inputs=3
  Trigonometric Function : Trigonometry
  Trigonometric Function1 : Trigonometry  Operator=cos
  Trigonometric Function2 : Trigonometry  Operator=cos
  Trigonometric Function3 : Trigonometry
  Trigonometric Function4 : Trigonometry
  Out1 : Outport  VectorParamsAs1DForOutWhenUnconnected=off
  wires:
  In8/1 -> Mux/3
  Integrator1/1 -> Out1/1
  1/m/1 -> Integrator/1
  Trigonometric Function4/1 -> Product1/2
  Integrator/1 -> Integrator1/1
  In7/1 -> Mux/2
  Add/1 -> Product2/1
  Product1/1 -> Add/2
  Product/1 -> Add/1
  In4/1 -> Trigonometric Function3/1
  Fcn/1 -> Product2/3
  Trigonometric Function1/1 -> Product/1
  In2/1 -> Trigonometric Function/1
  Trigonometric Function/1 -> Product/2
  Trigonometric Function2/1 -> Product/3
  Trigonometric Function3/1 -> Product1/1
  CT/1 -> Product2/2
  In1/1 -> Trigonometric Function1/1
  Product2/1 -> 1/m/1
  In3/1 -> Trigonometric Function2/1
  Mux/1 -> Fcn/1
  In6/1 -> Mux/1
  In5/1 -> Trigonometric Function4/1
  In9/1 -> Mux/4

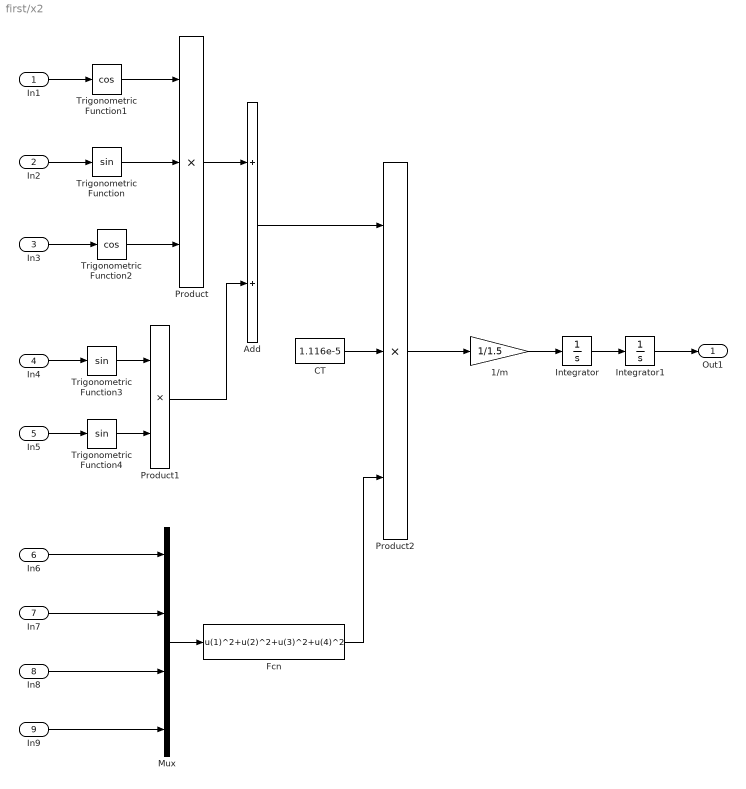
== system first/x2 ==
  In1 : Inport
  In2 : Inport  Port=2
  In3 : Inport  Port=3
  In4 : Inport  Port=4
  In5 : Inport  Port=5
  In6 : Inport  Port=6
  In7 : Inport  Port=7
  In8 : Inport  Port=8
  In9 : Inport  Port=9
  1/m : Gain  Gain=1/1.5
  Add : Sum
  CT : Constant  Value=1.116e-5
  Fcn : Fcn  Expr=u(1)^2+u(2)^2+u(3)^2+u(4)^2
  Integrator : Integrator
  Integrator1 : Integrator
  Mux : Mux
  Product : Product  Inputs=3
  Product1 : Product
  Product2 : Product  Inputs=3
  Trigonometric Function : Trigonometry
  Trigonometric Function1 : Trigonometry  Operator=cos
  Trigonometric Function2 : Trigonometry  Operator=cos
  Trigonometric Function3 : Trigonometry
  Trigonometric Function4 : Trigonometry
  Out1 : Outport  VectorParamsAs1DForOutWhenUnconnected=off
  wires:
  In8/1 -> Mux/3
  Integrator1/1 -> Out1/1
  1/m/1 -> Integrator/1
  Trigonometric Function4/1 -> Product1/2
  Integrator/1 -> Integrator1/1
  In7/1 -> Mux/2
  Add/1 -> Product2/1
  Product1/1 -> Add/2
  Product/1 -> Add/1
  In4/1 -> Trigonometric Function3/1
  Fcn/1 -> Product2/3
  Trigonometric Function1/1 -> Product/1
  In2/1 -> Trigonometric Function/1
  Trigonometric Function/1 -> Product/2
  Trigonometric Function2/1 -> Product/3
  Trigonometric Function3/1 -> Product1/1
  CT/1 -> Product2/2
  In1/1 -> Trigonometric Function1/1
  Product2/1 -> 1/m/1
  In3/1 -> Trigonometric Function2/1
  Mux/1 -> Fcn/1
  In6/1 -> Mux/1
  In5/1 -> Trigonometric Function4/1
  In9/1 -> Mux/4

== system first/x3 ==
  In1 : Inport
  In2 : Inport  Port=2
  In3 : Inport  Port=3
  In4 : Inport  Port=4
  In5 : Inport  Port=5
  In6 : Inport  Port=6
  In7 : Inport  Port=7
  In8 : Inport  Port=8
  In9 : Inport  Port=9
  1/m : Gain  Gain=1/1.5
  Add : Sum
  CT : Constant  Value=1.116e-5
  Fcn : Fcn  Expr=u(1)^2+u(2)^2+u(3)^2+u(4)^2
  Integrator : Integrator
  Integrator1 : Integrator
  Mux : Mux
  Product : Product  Inputs=3
  Product1 : Product
  Product2 : Product  Inputs=3
  Trigonometric Function : Trigonometry
  Trigonometric Function1 : Trigonometry  Operator=cos
  Trigonometric Function2 : Trigonometry  Operator=cos
  Trigonometric Function3 : Trigonometry
  Trigonometric Function4 : Trigonometry
  Out1 : Outport  VectorParamsAs1DForOutWhenUnconnected=off
  wires:
  In8/1 -> Mux/3
  Integrator1/1 -> Out1/1
  1/m/1 -> Integrator/1
  Trigonometric Function4/1 -> Product1/2
  Integrator/1 -> Integrator1/1
  In7/1 -> Mux/2
  Add/1 -> Product2/1
  Product1/1 -> Add/2
  Product/1 -> Add/1
  In4/1 -> Trigonometric Function3/1
  Fcn/1 -> Product2/3
  Trigonometric Function1/1 -> Product/1
  In2/1 -> Trigonometric Function/1
  Trigonometric Function/1 -> Product/2
  Trigonometric Function2/1 -> Product/3
  Trigonometric Function3/1 -> Product1/1
  CT/1 -> Product2/2
  In1/1 -> Trigonometric Function1/1
  Product2/1 -> 1/m/1
  In3/1 -> Trigonometric Function2/1
  Mux/1 -> Fcn/1
  In6/1 -> Mux/1
  In5/1 -> Trigonometric Function4/1
  In9/1 -> Mux/4

== system first/Attitude Control Module/Subsystem ==
  w2 : Inport
  w4 : Inport  Port=2
  In3 : Inport  Port=3
  In4 : Inport  Port=4
  1/Jxx : Gain  Gain=1/(1.745e-2)
  Add : Sum  Inputs=+-
  Add1 : Sum
  Add2 : Sum  Inputs=+-
  CT : Constant  Value=1.116e-5
  Fcn : Fcn  Expr=u(1)^2
  Fcn1 : Fcn  Expr=u(1)^2
  Jyy : Constant  Value=1.745e-2
  "Jzz " : Constant  Value=3.175e-2
  Product : Product
  Product1 : Product
  Product2 : Product  Inputs=3
  d : Constant  Value=0.225
  Out1 : Outport  VectorParamsAs1DForOutWhenUnconnected=off
  wires:
  Product2/1 -> Add1/1
  Fcn/1 -> Add2/2
  CT/1 -> Product2/3
  "Jzz "/1 -> Add/2
  Add1/1 -> 1/Jxx/1
  Fcn1/1 -> Add2/1
  Add2/1 -> Product2/1
  Product1/1 -> Add1/2
  Product/1 -> Product1/2
  d/1 -> Product2/2
  In4/1 -> Product/2
  Jyy/1 -> Add/1
  w4/1 -> Fcn/1
  Add/1 -> Product1/1
  1/Jxx/1 -> Out1/1
  w2/1 -> Fcn1/1
  In3/1 -> Product/1

== system first/Attitude Control Module/Subsystem1 ==
  w3 : Inport
  w1 : Inport  Port=2
  In3 : Inport  Port=3
  In4 : Inport  Port=4
  1/Jxx : Gain  Gain=1/(1.745e-2)
  Add : Sum  Inputs=+-
  Add1 : Sum
  Add2 : Sum  Inputs=+-
  CT : Constant  Value=1.116e-5
  Fcn : Fcn  Expr=u(1)^2
  Fcn1 : Fcn  Expr=u(1)^2
  Jxx : Constant  Value=1.745e-2
  Jzz : Constant  Value=3.175e-2
  Product : Product
  Product1 : Product
  Product2 : Product  Inputs=3
  d : Constant  Value=0.225
  Out1 : Outport  VectorParamsAs1DForOutWhenUnconnected=off
  wires:
  Product2/1 -> Add1/1
  Fcn/1 -> Add2/2
  CT/1 -> Product2/3
  Jxx/1 -> Add/2
  Add1/1 -> 1/Jxx/1
  Fcn1/1 -> Add2/1
  Add2/1 -> Product2/1
  Product1/1 -> Add1/2
  Product/1 -> Product1/2
  d/1 -> Product2/2
  In4/1 -> Product/2
  Jzz/1 -> Add/1
  w1/1 -> Fcn/1
  Add/1 -> Product1/1
  1/Jxx/1 -> Out1/1
  w3/1 -> Fcn1/1
  In3/1 -> Product/1

== system first/Attitude Control Module/Subsystem2 ==
  w1 : Inport
  w2 : Inport  Port=2
  In3 : Inport  Port=3
  In4 : Inport  Port=4
  w3 : Inport  Port=5
  w4 : Inport  Port=6
  1/Jxx : Gain  Gain=1/(3.175e-2)
  Add : Sum  Inputs=+-
  Add1 : Sum
  Add2 : Sum  Inputs=+-+-
  CM : Constant  Value=1.474e-7
  Fcn{,1..3} (4 alike) : Fcn  Expr=u(1)^2
  Jxx : Constant  Value=1.745e-2
  Jyy : Constant  Value=1.745e-2
  Product : Product
  Product1 : Product
  Product2 : Product
  Out1 : Outport  VectorParamsAs1DForOutWhenUnconnected=off
  wires:
  Product2/1 -> Add1/1
  CM/1 -> Product2/2
  Jyy/1 -> Add/2
  Add1/1 -> 1/Jxx/1
  Add2/1 -> Product2/1
  Product1/1 -> Add1/2
  Product/1 -> Product1/2
  In4/1 -> Product/2
  Jxx/1 -> Add/1
  Add/1 -> Product1/1
  1/Jxx/1 -> Out1/1
  In3/1 -> Product/1
  Fcn1/1 -> Add2/1
  Fcn/1 -> Add2/2
  Fcn3/1 -> Add2/3
  Fcn2/1 -> Add2/4
  w2/1 -> Fcn1/1
  w4/1 -> Fcn3/1
  w1/1 -> Fcn/1
  w3/1 -> Fcn2/1

== system first/Attitude Control Module1/Subsystem ==
  w2 : Inport
  w4 : Inport  Port=2
  In3 : Inport  Port=3
  In4 : Inport  Port=4
  1/Jxx : Gain  Gain=1/(1.745e-2)
  Add : Sum  Inputs=+-
  Add1 : Sum
  Add2 : Sum  Inputs=+-
  CT : Constant  Value=1.116e-5
  Fcn : Fcn  Expr=u(1)^2
  Fcn1 : Fcn  Expr=u(1)^2
  Jyy : Constant  Value=1.745e-2
  "Jzz " : Constant  Value=3.175e-2
  Product : Product
  Product1 : Product
  Product2 : Product  Inputs=3
  d : Constant  Value=0.225
  Out1 : Outport  VectorParamsAs1DForOutWhenUnconnected=off
  wires:
  Product2/1 -> Add1/1
  Fcn/1 -> Add2/2
  CT/1 -> Product2/3
  "Jzz "/1 -> Add/2
  Add1/1 -> 1/Jxx/1
  Fcn1/1 -> Add2/1
  Add2/1 -> Product2/1
  Product1/1 -> Add1/2
  Product/1 -> Product1/2
  d/1 -> Product2/2
  In4/1 -> Product/2
  Jyy/1 -> Add/1
  w4/1 -> Fcn/1
  Add/1 -> Product1/1
  1/Jxx/1 -> Out1/1
  w2/1 -> Fcn1/1
  In3/1 -> Product/1

== system first/Attitude Control Module1/Subsystem1 ==
  w3 : Inport
  w1 : Inport  Port=2
  In3 : Inport  Port=3
  In4 : Inport  Port=4
  1/Jxx : Gain  Gain=1/(1.745e-2)
  Add : Sum  Inputs=+-
  Add1 : Sum
  Add2 : Sum  Inputs=+-
  CT : Constant  Value=1.116e-5
  Fcn : Fcn  Expr=u(1)^2
  Fcn1 : Fcn  Expr=u(1)^2
  Jxx : Constant  Value=1.745e-2
  Jzz : Constant  Value=3.175e-2
  Product : Product
  Product1 : Product
  Product2 : Product  Inputs=3
  d : Constant  Value=0.225
  Out1 : Outport  VectorParamsAs1DForOutWhenUnconnected=off
  wires:
  Product2/1 -> Add1/1
  Fcn/1 -> Add2/2
  CT/1 -> Product2/3
  Jxx/1 -> Add/2
  Add1/1 -> 1/Jxx/1
  Fcn1/1 -> Add2/1
  Add2/1 -> Product2/1
  Product1/1 -> Add1/2
  Product/1 -> Product1/2
  d/1 -> Product2/2
  In4/1 -> Product/2
  Jzz/1 -> Add/1
  w1/1 -> Fcn/1
  Add/1 -> Product1/1
  1/Jxx/1 -> Out1/1
  w3/1 -> Fcn1/1
  In3/1 -> Product/1

== system first/Attitude Control Module1/Subsystem2 ==
  w1 : Inport
  w2 : Inport  Port=2
  In3 : Inport  Port=3
  In4 : Inport  Port=4
  w3 : Inport  Port=5
  w4 : Inport  Port=6
  1/Jxx : Gain  Gain=1/(3.175e-2)
  Add : Sum  Inputs=+-
  Add1 : Sum
  Add2 : Sum  Inputs=+-+-
  CM : Constant  Value=1.474e-7
  Fcn{,1..3} (4 alike) : Fcn  Expr=u(1)^2
  Jxx : Constant  Value=1.745e-2
  Jyy : Constant  Value=1.745e-2
  Product : Product
  Product1 : Product
  Product2 : Product
  Out1 : Outport  VectorParamsAs1DForOutWhenUnconnected=off
  wires:
  Product2/1 -> Add1/1
  CM/1 -> Product2/2
  Jyy/1 -> Add/2
  Add1/1 -> 1/Jxx/1
  Add2/1 -> Product2/1
  Product1/1 -> Add1/2
  Product/1 -> Product1/2
  In4/1 -> Product/2
  Jxx/1 -> Add/1
  Add/1 -> Product1/1
  1/Jxx/1 -> Out1/1
  In3/1 -> Product/1
  Fcn1/1 -> Add2/1
  Fcn/1 -> Add2/2
  Fcn3/1 -> Add2/3
  Fcn2/1 -> Add2/4
  w2/1 -> Fcn1/1
  w4/1 -> Fcn3/1
  w1/1 -> Fcn/1
  w3/1 -> Fcn2/1

== system first/Attitude Control Module2/Subsystem ==
  w2 : Inport
  w4 : Inport  Port=2
  In3 : Inport  Port=3
  In4 : Inport  Port=4
  1/Jxx : Gain  Gain=1/(1.745e-2)
  Add : Sum  Inputs=+-
  Add1 : Sum
  Add2 : Sum  Inputs=+-
  CT : Constant  Value=1.116e-5
  Fcn : Fcn  Expr=u(1)^2
  Fcn1 : Fcn  Expr=u(1)^2
  Jyy : Constant  Value=1.745e-2
  "Jzz " : Constant  Value=3.175e-2
  Product : Product
  Product1 : Product
  Product2 : Product  Inputs=3
  d : Constant  Value=0.225
  Out1 : Outport  VectorParamsAs1DForOutWhenUnconnected=off
  wires:
  Product2/1 -> Add1/1
  Fcn/1 -> Add2/2
  CT/1 -> Product2/3
  "Jzz "/1 -> Add/2
  Add1/1 -> 1/Jxx/1
  Fcn1/1 -> Add2/1
  Add2/1 -> Product2/1
  Product1/1 -> Add1/2
  Product/1 -> Product1/2
  d/1 -> Product2/2
  In4/1 -> Product/2
  Jyy/1 -> Add/1
  w4/1 -> Fcn/1
  Add/1 -> Product1/1
  1/Jxx/1 -> Out1/1
  w2/1 -> Fcn1/1
  In3/1 -> Product/1

== system first/Attitude Control Module2/Subsystem1 ==
  w3 : Inport
  w1 : Inport  Port=2
  In3 : Inport  Port=3
  In4 : Inport  Port=4
  1/Jxx : Gain  Gain=1/(1.745e-2)
  Add : Sum  Inputs=+-
  Add1 : Sum
  Add2 : Sum  Inputs=+-
  CT : Constant  Value=1.116e-5
  Fcn : Fcn  Expr=u(1)^2
  Fcn1 : Fcn  Expr=u(1)^2
  Jxx : Constant  Value=1.745e-2
  Jzz : Constant  Value=3.175e-2
  Product : Product
  Product1 : Product
  Product2 : Product  Inputs=3
  d : Constant  Value=0.225
  Out1 : Outport  VectorParamsAs1DForOutWhenUnconnected=off
  wires:
  Product2/1 -> Add1/1
  Fcn/1 -> Add2/2
  CT/1 -> Product2/3
  Jxx/1 -> Add/2
  Add1/1 -> 1/Jxx/1
  Fcn1/1 -> Add2/1
  Add2/1 -> Product2/1
  Product1/1 -> Add1/2
  Product/1 -> Product1/2
  d/1 -> Product2/2
  In4/1 -> Product/2
  Jzz/1 -> Add/1
  w1/1 -> Fcn/1
  Add/1 -> Product1/1
  1/Jxx/1 -> Out1/1
  w3/1 -> Fcn1/1
  In3/1 -> Product/1

== system first/Attitude Control Module2/Subsystem2 ==
  w1 : Inport
  w2 : Inport  Port=2
  In3 : Inport  Port=3
  In4 : Inport  Port=4
  w3 : Inport  Port=5
  w4 : Inport  Port=6
  1/Jxx : Gain  Gain=1/(3.175e-2)
  Add : Sum  Inputs=+-
  Add1 : Sum
  Add2 : Sum  Inputs=+-+-
  CM : Constant  Value=1.474e-7
  Fcn{,1..3} (4 alike) : Fcn  Expr=u(1)^2
  Jxx : Constant  Value=1.745e-2
  Jyy : Constant  Value=1.745e-2
  Product : Product
  Product1 : Product
  Product2 : Product
  Out1 : Outport  VectorParamsAs1DForOutWhenUnconnected=off
  wires:
  Product2/1 -> Add1/1
  CM/1 -> Product2/2
  Jyy/1 -> Add/2
  Add1/1 -> 1/Jxx/1
  Add2/1 -> Product2/1
  Product1/1 -> Add1/2
  Product/1 -> Product1/2
  In4/1 -> Product/2
  Jxx/1 -> Add/1
  Add/1 -> Product1/1
  1/Jxx/1 -> Out1/1
  In3/1 -> Product/1
  Fcn1/1 -> Add2/1
  Fcn/1 -> Add2/2
  Fcn3/1 -> Add2/3
  Fcn2/1 -> Add2/4
  w2/1 -> Fcn1/1
  w4/1 -> Fcn3/1
  w1/1 -> Fcn/1
  w3/1 -> Fcn2/1

== system first/Attitude Control Module3/Subsystem ==
  w2 : Inport
  w4 : Inport  Port=2
  In3 : Inport  Port=3
  In4 : Inport  Port=4
  1/Jxx : Gain  Gain=1/(1.745e-2)
  Add : Sum  Inputs=+-
  Add1 : Sum
  Add2 : Sum  Inputs=+-
  CT : Constant  Value=1.116e-5
  Fcn : Fcn  Expr=u(1)^2
  Fcn1 : Fcn  Expr=u(1)^2
  Jyy : Constant  Value=1.745e-2
  "Jzz " : Constant  Value=3.175e-2
  Product : Product
  Product1 : Product
  Product2 : Product  Inputs=3
  d : Constant  Value=0.225
  Out1 : Outport  VectorParamsAs1DForOutWhenUnconnected=off
  wires:
  Product2/1 -> Add1/1
  Fcn/1 -> Add2/2
  CT/1 -> Product2/3
  "Jzz "/1 -> Add/2
  Add1/1 -> 1/Jxx/1
  Fcn1/1 -> Add2/1
  Add2/1 -> Product2/1
  Product1/1 -> Add1/2
  Product/1 -> Product1/2
  d/1 -> Product2/2
  In4/1 -> Product/2
  Jyy/1 -> Add/1
  w4/1 -> Fcn/1
  Add/1 -> Product1/1
  1/Jxx/1 -> Out1/1
  w2/1 -> Fcn1/1
  In3/1 -> Product/1

== system first/Attitude Control Module3/Subsystem1 ==
  w3 : Inport
  w1 : Inport  Port=2
  In3 : Inport  Port=3
  In4 : Inport  Port=4
  1/Jxx : Gain  Gain=1/(1.745e-2)
  Add : Sum  Inputs=+-
  Add1 : Sum
  Add2 : Sum  Inputs=+-
  CT : Constant  Value=1.116e-5
  Fcn : Fcn  Expr=u(1)^2
  Fcn1 : Fcn  Expr=u(1)^2
  Jxx : Constant  Value=1.745e-2
  Jzz : Constant  Value=3.175e-2
  Product : Product
  Product1 : Product
  Product2 : Product  Inputs=3
  d : Constant  Value=0.225
  Out1 : Outport  VectorParamsAs1DForOutWhenUnconnected=off
  wires:
  Product2/1 -> Add1/1
  Fcn/1 -> Add2/2
  CT/1 -> Product2/3
  Jxx/1 -> Add/2
  Add1/1 -> 1/Jxx/1
  Fcn1/1 -> Add2/1
  Add2/1 -> Product2/1
  Product1/1 -> Add1/2
  Product/1 -> Product1/2
  d/1 -> Product2/2
  In4/1 -> Product/2
  Jzz/1 -> Add/1
  w1/1 -> Fcn/1
  Add/1 -> Product1/1
  1/Jxx/1 -> Out1/1
  w3/1 -> Fcn1/1
  In3/1 -> Product/1

== system first/Attitude Control Module3/Subsystem2 ==
  w1 : Inport
  w2 : Inport  Port=2
  In3 : Inport  Port=3
  In4 : Inport  Port=4
  w3 : Inport  Port=5
  w4 : Inport  Port=6
  1/Jxx : Gain  Gain=1/(3.175e-2)
  Add : Sum  Inputs=+-
  Add1 : Sum
  Add2 : Sum  Inputs=+-+-
  CM : Constant  Value=1.474e-7
  Fcn{,1..3} (4 alike) : Fcn  Expr=u(1)^2
  Jxx : Constant  Value=1.745e-2
  Jyy : Constant  Value=1.745e-2
  Product : Product
  Product1 : Product
  Product2 : Product
  Out1 : Outport  VectorParamsAs1DForOutWhenUnconnected=off
  wires:
  Product2/1 -> Add1/1
  CM/1 -> Product2/2
  Jyy/1 -> Add/2
  Add1/1 -> 1/Jxx/1
  Add2/1 -> Product2/1
  Product1/1 -> Add1/2
  Product/1 -> Product1/2
  In4/1 -> Product/2
  Jxx/1 -> Add/1
  Add/1 -> Product1/1
  1/Jxx/1 -> Out1/1
  In3/1 -> Product/1
  Fcn1/1 -> Add2/1
  Fcn/1 -> Add2/2
  Fcn3/1 -> Add2/3
  Fcn2/1 -> Add2/4
  w2/1 -> Fcn1/1
  w4/1 -> Fcn3/1
  w1/1 -> Fcn/1
  w3/1 -> Fcn2/1
